simulink model "DrivetrainHevP2_SSC"  (R2022a)
settings: Solver=daessc  StartTime=0.0  StopTime=100  RelTol=1e-3
model workspace (MAT data in the model file):
  Aeff = 0.0314159265359
  Af = 2.27
  Apist_C0 = 0.0314159265359
  Apist_TCC = 0.001
  Bx = 10
  Cd = 0.25
  CoulFr_ShaftIn = 0
  Cx = 1.9
  DensAir = 1.293
  DerFac_C0 = 1
  DerFac_TCC = 1
  Drag_C0 = 0
  Drag_TCC = 0
  Dx = 1
  Eff_Diff = [0.98 0.98]
  Ex = 0.97
  FDrive = 3.32
  FZMAX = 6570
  FZMIN = 0
  G = [0 1 2 3 4 5 6]
  G_o = 1
  Iyy = 0.8
  Iyy_Whl = 0.8
  JCa_Diff = 0.001
  JEng = 0.01
  JMot = 0.21
  JPl_Diff = 0.001
  JShIn = 1e-05
  JShOut = 0.15
  Jd = 0.025
  Ji = 0.21
  Jin_Cltch = 0.2
  Jout = [0.009 0.01 0.01 0.01 0.01 0.01 0.01]
  Jout_Cltch = 0.01
  Jt = 0.01
  Jw1 = 0.01
  Jw2 = 0.01
  K_c = 10000
  KinFr_C0 = 0.4
  KinFr_TCC = 0.3
  Lrel = 0.15
  Mass = 1623
  N = [0.001 4.212 2.637 1.8 1.386 1 0.772]
  NF = 2
  NR = 2
  Ndiff = 3.32
  Ndisk = 1
  Neff_C0 = 1
  Neff_TCC = 6
  PEng_C0 = 30000
  PEng_TCC = 100
  Pabs = 101325
  Press = 300000
  PwrThr_Diff = [0.001 0.001]
  RatFr_ShaftIn = 1.1
  Re = 0.327
  Reff = 0.11
  Reff_C0 = 0.11
  Reff_TCC = 130
  Rm = 0.15
  SprStff_ShaftIn = 10000
  StatFr_C0 = 0.45
  StatFr_TCC = 0.35
  T = 273
  Temp_bpts = [313 358]
  Trq_bpts = [25 50 75 100 150 200 250]
  UNLOADED_RADIUS = 0.336
  VXLOW = 2
  VisFr_Diff = [0.001 0.001]
  ViscFr_ShaftIn = 400
  aMy = 0.01
  a_CG = 1.09
  alphaMy = 0
  b : Simulink.Parameter (value not decoded)
  bMy = 0
  b_CG = 1.7
  bd = 0.001
  betaMy = 1
  bi = 0.001
  bin_Cltch = 0.003
  bout = [0.003 0.003 0.003 0.003 0.003 0.003 0.003]
  bout_Cltch = 0.003
  br = 0.001
  bt = 0.001
  bw1 = 0.001
  bw2 = 0.001
  cMy = 0
  disk_abore = 0.05
  domega_o = 0
  eta = [0.95 0.95 0.95 0.95 0.95 0.95 0.95]
  eta_diff = 0.98
  eta_tbl = [1 1 1 1 1 1 1 1 1 1 1 1 ... (1078 elements, 7x11x7x2)]
  g = 9.81
  h = 0.5
  k : Simulink.Parameter (value not decoded)
  kappamax = 1.5
  lam_x = 1
  mu_kinetic = 0.35
  mu_static = 0.45
  muk = 0.4
  mus = 0.45
  num_pads = 2
  omega_bpts = [500.383141081 749.619781963 1002.67614148 1250.9578527 1499.23956393 1747.52127515 1995.80298637 2501.9157054 2998.47912785 4001.15526933 5003.83141081]
  omega_c : Simulink.Parameter (value not decoded)
  omega_o = 0
  omegai_o = 0
  omegal = 94.2477796077
  omegao = 0
  omegat_o = 0
  omegau = 83.7758040957
  omegaw1o = 0
  omegaw2o = 0
  phi = [0 0.5 0.6 0.7 0.8 0.87 0.92 0.94 0.96 0.97]
  phi_new = [0 0.5 0.6 0.7 0.8 0.87 0.92 0.94 0.96 0.97 0.99 1.02 ... (16 elements, 1x16)]
  philu = 0.85
  press = 700000
  psi = [12.2938 12.8588 13.1452 13.6285 14.6163 16.2675 19.3503 22.1046 29.9986 50]
  psi_new = [12.2938 12.8588 13.1452 13.6285 14.6163 16.2675 19.3503 22.1046 29.9986 50 48 41.76 ... (16 elements, 1x16)]
  tauC = 0.25
  tauTC = 0.1
  tau_s = 0.1
  theta_o = 0
  wc = 10
  win_o = 0
  wout_o = 0
  x_o = 0
  xdot_o = 0
  zeta = [2.232 1.5462 1.4058 1.2746 1.1528 1.0732 1.0192 0.9983 0.9983 0.9983]
  zeta_new = [2.232 1.5462 1.4058 1.2746 1.1528 1.0732 1.0192 0.9983 0.9983 0.9983 0.979797979798 1.04382929642 ... (16 elements, 1x16)]
libraries: fl_lib x66, nesl_utility x40, sdl_lib x25, simulink x7, autolibpowerinfoutils x5
(part 2 of 3)

== system DrivetrainHevP2_SSC/Sensor3 ==
  DiffTQ : nesl_utility/PS-Simulink Converter  PhysicalDomain=network_engine_domain  SubClassName=ps_output  LeftPortType=input  RightPortType=output  PseudoPeriodic=off  Frequencies=[]  VectorFormat=1-D array  Unit=1  AffineConversion=off
      settings: SourceProductBaseCode=SS,PW,VE
  Ideal Rotational Motion Sensor : fl_lib/Mechanical/Mechanical Sensors/Ideal Rotational Motion Sensor  wrap_angle=simscape.enum.onoff.off  offset=0 rad
      settings: SourceProductBaseCode=PW,SS,VE
  Ideal Torque Sensor : fl_lib/Mechanical/Mechanical Sensors/Ideal Torque Sensor
      settings: SourceProductBaseCode=PW,SS,VE
  Mechanical Rotational Reference : fl_lib/Mechanical/Rotational Elements/Mechanical Rotational Reference
      settings: SourceProductBaseCode=PW,SS,VE
  PS Terminator : fl_lib/Physical Signals/Sinks/PS Terminator
      settings: SourceProductBaseCode=PW,SS,VE
  PS-Simulink Converter : nesl_utility/PS-Simulink Converter  PhysicalDomain=network_engine_domain  SubClassName=ps_output  LeftPortType=input  RightPortType=output  PseudoPeriodic=off  Frequencies=[]  VectorFormat=1-D array  Unit=inherit  AffineConversion=off
      settings: SourceProductBaseCode=SS,PW,VE
  R : PMIOPort  Side=Left
  C : PMIOPort  Port=2  Side=Right
  Trq : Outport
  Spd : Outport  Port=2
  wires:
  DiffTQ/1 -> Trq/1
  PS-Simulink Converter/1 -> Spd/1
  connections:
  DiffTQ/LConn1 -- Ideal Torque Sensor/RConn2
  Ideal Torque Sensor/RConn1 -- C/RConn1
  Ideal Torque Sensor/LConn1 -- R/RConn1 -- Ideal Rotational Motion Sensor/LConn1
  PS Terminator/LConn1 -- Ideal Rotational Motion Sensor/RConn3
  PS-Simulink Converter/LConn1 -- Ideal Rotational Motion Sensor/RConn2
  Mechanical Rotational Reference/LConn1 -- Ideal Rotational Motion Sensor/RConn1

== system DrivetrainHevP2_SSC/Sensor4 ==
  Force : nesl_utility/PS-Simulink Converter  PhysicalDomain=network_engine_domain  SubClassName=ps_output  LeftPortType=input  RightPortType=output  PseudoPeriodic=off  Frequencies=[]  VectorFormat=1-D array  Unit=1  AffineConversion=off
      settings: SourceProductBaseCode=SS,PW,VE
  Ideal Force Sensor : fl_lib/Mechanical/Mechanical Sensors/Ideal Force Sensor
      settings: SourceProductBaseCode=PW,SS,VE
  Ideal Translational Motion Sensor : fl_lib/Mechanical/Mechanical Sensors/Ideal Translational Motion Sensor  offset=0 m
      settings: SourceProductBaseCode=PW,SS,VE
  Mechanical Translational Reference : fl_lib/Mechanical/Translational Elements/Mechanical Translational Reference
      settings: SourceProductBaseCode=PW,SS,VE
  SPD : nesl_utility/PS-Simulink Converter  PhysicalDomain=network_engine_domain  SubClassName=ps_output  LeftPortType=input  RightPortType=output  PseudoPeriodic=off  Frequencies=[]  VectorFormat=1-D array  Unit=1  AffineConversion=off
      settings: SourceProductBaseCode=SS,PW,VE
  Out : PMIOPort  Side=Left
  H : PMIOPort  Port=2  Side=Right
  VEVspd : Outport
  VEHforce : Outport  Port=2
  wires:
  Force/1 -> VEHforce/1
  SPD/1 -> VEVspd/1
  connections:
  Ideal Force Sensor/RConn1 -- Out/RConn1
  Ideal Force Sensor/RConn2 -- Force/LConn1
  SPD/LConn1 -- Ideal Translational Motion Sensor/RConn2
  Ideal Force Sensor/LConn1 -- Ideal Translational Motion Sensor/LConn1 -- H/RConn1
  Mechanical Translational Reference/LConn1 -- Ideal Translational Motion Sensor/RConn1

== system DrivetrainHevP2_SSC/Torque Converter and Lockup Clutch ==
  MtrTrq : Inport
  ClutchTrq : Inport  Port=2
  ClutchSpd : Inport  Port=3
  MtrSpd : Inport  Port=4
  TurbTrq : Inport  Port=5
  TurbSpd : Inport  Port=6
  Power Accounting Bus Creator2 : autolibpowerinfoutils/Power Accounting Bus Creator  AssctBlkSelPopup=Parent  RefBlkName='diff'  PwrTrnsfrdCheckBox=on  PwrNotTrnsfrdCheckBox=on  PwrStoredCheckBox=on  aMode=aMode
      settings: SourceProductBaseCode=PW,DR,MT,VE
  PwrAccountingDiff : Subsystem
  Terminator5 : Terminator
  wires:
  TurbTrq/1 -> PwrAccountingDiff/3(TurbTrq)
  TurbSpd/1 -> PwrAccountingDiff/5(TurbSpd)
  MtrTrq/1 -> PwrAccountingDiff/4(MtrTrq)
  ClutchTrq/1 -> PwrAccountingDiff/2(ClutchTrq)
  PwrAccountingDiff/3(PWRstored) -> Power Accounting Bus Creator2/3
  PwrAccountingDiff/1(PwrTrnsfrd) -> Power Accounting Bus Creator2/1
  PwrAccountingDiff/2(PwrNotTrnsfrd) -> Power Accounting Bus Creator2/2
  Power Accounting Bus Creator2/1 -> Terminator5/1
  ClutchSpd/1 -> PwrAccountingDiff/1(ClutchSpd)
  MtrSpd/1 -> PwrAccountingDiff/6(MtrSpd)

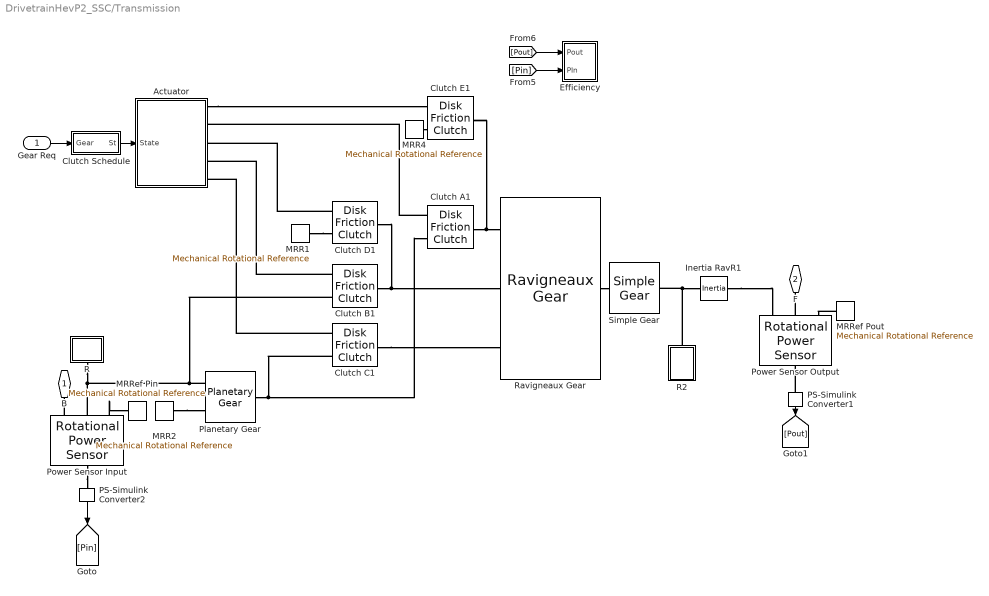
== system DrivetrainHevP2_SSC/Transmission ==
  Gear Req : Inport
  Actuator : Subsystem
  Clutch Schedule : Subsystem
  Clutch A1 : sdl_lib/Clutches/Disk Friction Clutch  geometry_model=sdl.enum.friction_geometry.annular  r_eff=130 mm  d_o=150 mm  d_i=100 mm  nS=6  piston_area=0.001 m^2  unidirectional=sdl.enum.directionality.bidirectional  friction_model=sdl.enum.friction_model_TLU_thermal.fixed  mu_w_vector=[ 0 0.1 0.2 0.3 0.4 0.5 1 2 5 10 100 1000 ] rad/s  temperature_TLU=[280.0, 300.0, 320.0] K  mu_static=0.65  mu_static_vector=[0.4, 0.38, 0.36]  mu_coulomb=0.6  mu_coulomb_vector=[ 0.29 0.28 0.26 0.22 0.21 0.2 0.2 0.19 0.19 0.19 0.19 0.19 ]  mu_coulomb_temp_vector=[0.3, 0.28, 0.25]  mu_coulomb_matrix=[0.34, 0.32, 0.3; 0.3, 0.28, 0.25; 0.25, 0.2, 0.15]  mu_interp_method=simscape.enum.interpolation.linear  mu_extrap_method=simscape.enum.extrapolation.linear  d_f=1  w_tol=0.001 rad/s  pressure_min=100 Pa  mu_visc=0 N*m/(rad/s)  initial_state_locked=sdl.enum.initial_lock.locked  enable_faults=simscape.enum.onoff.off  fault_type=sdl.enum.clutchFault.lock  external_fault=simscape.enum.onoff.off  temporal_fault=simscape.enum.onoff.off  fault_time=5 s  report_fault=simscape.enum.assert.action.none  thermal_mass=25 kJ/K  T_init=300 K
      settings: SourceProductBaseCode=LD  InternalSimscapePortConfiguration="{\"Bottom\":[],\"Left\":[{\"id\":\"P\",\"label\":\"P\",\"type\":\"input\"},{\"id\":\"B\",\"label\":\"B\",\"type\":\"foundation.mechanical.rotational.rotational\"}],\"Right\":[{\"id\":\"F\",\"label\":\"F\",\"type\":\"foundation.mechanical.rotational.rotational\"}],\"Top\":[]}"
  Clutch B1 : sdl_lib/Clutches/Disk Friction Clutch  geometry_model=sdl.enum.friction_geometry.annular  r_eff=130 mm  d_o=150 mm  d_i=100 mm  nS=6  piston_area=0.001 m^2  unidirectional=sdl.enum.directionality.bidirectional  friction_model=sdl.enum.friction_model_TLU_thermal.fixed  mu_w_vector=[ 0 0.1 0.2 0.3 0.4 0.5 1 2 5 10 100 1000 ] rad/s  temperature_TLU=[280.0, 300.0, 320.0] K  mu_static=0.65  mu_static_vector=[0.4, 0.38, 0.36]  mu_coulomb=0.6  mu_coulomb_vector=[ 0.29 0.28 0.26 0.22 0.21 0.2 0.2 0.19 0.19 0.19 0.19 0.19 ]  mu_coulomb_temp_vector=[0.3, 0.28, 0.25]  mu_coulomb_matrix=[0.34, 0.32, 0.3; 0.3, 0.28, 0.25; 0.25, 0.2, 0.15]  mu_interp_method=simscape.enum.interpolation.linear  mu_extrap_method=simscape.enum.extrapolation.linear  d_f=1  w_tol=0.001 rad/s  pressure_min=100 Pa  mu_visc=0 N*m/(rad/s)  initial_state_locked=sdl.enum.initial_lock.unlocked  enable_faults=simscape.enum.onoff.off  fault_type=sdl.enum.clutchFault.lock  external_fault=simscape.enum.onoff.off  temporal_fault=simscape.enum.onoff.off  fault_time=5 s  report_fault=simscape.enum.assert.action.none  thermal_mass=25 kJ/K  T_init=300 K
      settings: SourceProductBaseCode=LD  InternalSimscapePortConfiguration="{\"Bottom\":[],\"Left\":[{\"id\":\"P\",\"label\":\"P\",\"type\":\"input\"},{\"id\":\"B\",\"label\":\"B\",\"type\":\"foundation.mechanical.rotational.rotational\"}],\"Right\":[{\"id\":\"F\",\"label\":\"F\",\"type\":\"foundation.mechanical.rotational.rotational\"}],\"Top\":[]}"
  Clutch C1 : sdl_lib/Clutches/Disk Friction Clutch  geometry_model=sdl.enum.friction_geometry.annular  r_eff=130 mm  d_o=150 mm  d_i=100 mm  nS=6  piston_area=0.001 m^2  unidirectional=sdl.enum.directionality.bidirectional  friction_model=sdl.enum.friction_model_TLU_thermal.fixed  mu_w_vector=[ 0 0.1 0.2 0.3 0.4 0.5 1 2 5 10 100 1000 ] rad/s  temperature_TLU=[280.0, 300.0, 320.0] K  mu_static=0.65  mu_static_vector=[0.4, 0.38, 0.36]  mu_coulomb=0.6  mu_coulomb_vector=[ 0.29 0.28 0.26 0.22 0.21 0.2 0.2 0.19 0.19 0.19 0.19 0.19 ]  mu_coulomb_temp_vector=[0.3, 0.28, 0.25]  mu_coulomb_matrix=[0.34, 0.32, 0.3; 0.3, 0.28, 0.25; 0.25, 0.2, 0.15]  mu_interp_method=simscape.enum.interpolation.linear  mu_extrap_method=simscape.enum.extrapolation.linear  d_f=1  w_tol=0.001 rad/s  pressure_min=100 Pa  mu_visc=0 N*m/(rad/s)  initial_state_locked=sdl.enum.initial_lock.unlocked  enable_faults=simscape.enum.onoff.off  fault_type=sdl.enum.clutchFault.lock  external_fault=simscape.enum.onoff.off  temporal_fault=simscape.enum.onoff.off  fault_time=5 s  report_fault=simscape.enum.assert.action.none  thermal_mass=25 kJ/K  T_init=300 K
      settings: SourceProductBaseCode=LD  InternalSimscapePortConfiguration="{\"Bottom\":[],\"Left\":[{\"id\":\"P\",\"label\":\"P\",\"type\":\"input\"},{\"id\":\"B\",\"label\":\"B\",\"type\":\"foundation.mechanical.rotational.rotational\"}],\"Right\":[{\"id\":\"F\",\"label\":\"F\",\"type\":\"foundation.mechanical.rotational.rotational\"}],\"Top\":[]}"
  Clutch D1 : sdl_lib/Clutches/Disk Friction Clutch  geometry_model=sdl.enum.friction_geometry.annular  r_eff=130 mm  d_o=150 mm  d_i=100 mm  nS=6  piston_area=0.001 m^2  unidirectional=sdl.enum.directionality.bidirectional  friction_model=sdl.enum.friction_model_TLU_thermal.fixed  mu_w_vector=[ 0 0.1 0.2 0.3 0.4 0.5 1 2 5 10 100 1000 ] rad/s  temperature_TLU=[280.0, 300.0, 320.0] K  mu_static=0.65  mu_static_vector=[0.4, 0.38, 0.36]  mu_coulomb=0.6  mu_coulomb_vector=[ 0.29 0.28 0.26 0.22 0.21 0.2 0.2 0.19 0.19 0.19 0.19 0.19 ]  mu_coulomb_temp_vector=[0.3, 0.28, 0.25]  mu_coulomb_matrix=[0.34, 0.32, 0.3; 0.3, 0.28, 0.25; 0.25, 0.2, 0.15]  mu_interp_method=simscape.enum.interpolation.linear  mu_extrap_method=simscape.enum.extrapolation.linear  d_f=1  w_tol=0.001 rad/s  pressure_min=100 Pa  mu_visc=0 N*m/(rad/s)  initial_state_locked=sdl.enum.initial_lock.locked  enable_faults=simscape.enum.onoff.off  fault_type=sdl.enum.clutchFault.lock  external_fault=simscape.enum.onoff.off  temporal_fault=simscape.enum.onoff.off  fault_time=5 s  report_fault=simscape.enum.assert.action.none  thermal_mass=25 kJ/K  T_init=300 K
      settings: SourceProductBaseCode=LD  InternalSimscapePortConfiguration="{\"Bottom\":[],\"Left\":[{\"id\":\"P\",\"label\":\"P\",\"type\":\"input\"},{\"id\":\"B\",\"label\":\"B\",\"type\":\"foundation.mechanical.rotational.rotational\"}],\"Right\":[{\"id\":\"F\",\"label\":\"F\",\"type\":\"foundation.mechanical.rotational.rotational\"}],\"Top\":[]}"
  Clutch E1 : sdl_lib/Clutches/Disk Friction Clutch  geometry_model=sdl.enum.friction_geometry.annular  r_eff=130 mm  d_o=150 mm  d_i=100 mm  nS=6  piston_area=0.001 m^2  unidirectional=sdl.enum.directionality.bidirectional  friction_model=sdl.enum.friction_model_TLU_thermal.fixed  mu_w_vector=[ 0 0.1 0.2 0.3 0.4 0.5 1 2 5 10 100 1000 ] rad/s  temperature_TLU=[280.0, 300.0, 320.0] K  mu_static=0.65  mu_static_vector=[0.4, 0.38, 0.36]  mu_coulomb=0.6  mu_coulomb_vector=[ 0.29 0.28 0.26 0.22 0.21 0.2 0.2 0.19 0.19 0.19 0.19 0.19 ]  mu_coulomb_temp_vector=[0.3, 0.28, 0.25]  mu_coulomb_matrix=[0.34, 0.32, 0.3; 0.3, 0.28, 0.25; 0.25, 0.2, 0.15]  mu_interp_method=simscape.enum.interpolation.linear  mu_extrap_method=simscape.enum.extrapolation.linear  d_f=1  w_tol=0.001 rad/s  pressure_min=100 Pa  mu_visc=0 N*m/(rad/s)  initial_state_locked=sdl.enum.initial_lock.unlocked  enable_faults=simscape.enum.onoff.off  fault_type=sdl.enum.clutchFault.lock  external_fault=simscape.enum.onoff.off  temporal_fault=simscape.enum.onoff.off  fault_time=5 s  report_fault=simscape.enum.assert.action.none  thermal_mass=25 kJ/K  T_init=300 K
      settings: SourceProductBaseCode=LD  InternalSimscapePortConfiguration="{\"Bottom\":[],\"Left\":[{\"id\":\"P\",\"label\":\"P\",\"type\":\"input\"},{\"id\":\"B\",\"label\":\"B\",\"type\":\"foundation.mechanical.rotational.rotational\"}],\"Right\":[{\"id\":\"F\",\"label\":\"F\",\"type\":\"foundation.mechanical.rotational.rotational\"}],\"Top\":[]}"
  Efficiency : Subsystem
  Inertia RavR1 : fl_lib/Mechanical/Rotational Elements/Inertia  inertia=0.01 kg*m^2  num_ports=foundation.enum.numPorts2.two  w_specify=on  w_priority=High  w=0 rad/s  w_nominal_specify=off  w_nominal_unit=rad/s  w_nominal_value=1  t_specify=off  t_priority=High  t=0 N*m  t_nominal_specify=off  t_nominal_unit=N*m  t_nominal_value=1
      settings: SourceProductBaseCode=PW,SS,VE  InternalSimscapePortConfiguration="{\"Bottom\":[],\"Left\":[{\"id\":\"I\",\"label\":\"\",\"type\":\"foundation.mechanical.rotational.rotational\"}],\"Right\":[{\"id\":\"J\",\"label\":\"\",\"type\":\"foundation.mechanical.rotational.rotational\"}],\"Top\":[]}"
  MRR1 : fl_lib/Mechanical/Rotational Elements/Mechanical Rotational Reference
      settings: SourceProductBaseCode=PW,SS,VE
  MRR2 : fl_lib/Mechanical/Rotational Elements/Mechanical Rotational Reference
      settings: SourceProductBaseCode=PW,SS,VE
  MRR4 : fl_lib/Mechanical/Rotational Elements/Mechanical Rotational Reference
      settings: SourceProductBaseCode=PW,SS,VE
  MRRef Pin : fl_lib/Mechanical/Rotational Elements/Mechanical Rotational Reference
      settings: SourceProductBaseCode=PW,SS,VE
  MRRef Pout : fl_lib/Mechanical/Rotational Elements/Mechanical Rotational Reference
      settings: SourceProductBaseCode=PW,SS,VE
  PS-Simulink Converter1 : nesl_utility/PS-Simulink Converter  PhysicalDomain=network_engine_domain  SubClassName=ps_output  LeftPortType=input  RightPortType=output  PseudoPeriodic=off  Frequencies=[]  VectorFormat=1-D array  Unit=HP_DIN  AffineConversion=off
      settings: SourceProductBaseCode=SS,PW,VE
  PS-Simulink Converter2 : nesl_utility/PS-Simulink Converter  PhysicalDomain=network_engine_domain  SubClassName=ps_output  LeftPortType=input  RightPortType=output  PseudoPeriodic=off  Frequencies=[]  VectorFormat=1-D array  Unit=HP_DIN  AffineConversion=off
      settings: SourceProductBaseCode=SS,PW,VE
  Planetary Gear : sdl_lib/Gears/Planetary Gear  rs_ratio=1.92424631  friction_model=sdl.enum.gear_friction.constant  efficiency=[ 0.95 0.95]  temperature_TLU=[ 280 300 320 ] K  efficiency_sp_TLU=[ 0.95 0.9 0.85 ]  efficiency_rp_TLU=[ 0.95 0.9 0.85 ]  pwr_thr=[ 0.001 0.001 ] W  mu_visc=[ 0 0 ] N*m/(rad/s)  model_inertia=simscape.enum.onoff.on  planet_inertia=0.001 kg*m^2  thermal_mass=50 J/K  T_init=300 K
      settings: SourceProductBaseCode=LD
  Power Sensor Input : sdl_lib/Sensors/Rotational Power Sensor  measurement_type=1  averaging_period=1 s  max_frequency=1000 Hz  max_speed=1000 rpm
      settings: SourceProductBaseCode=LD  InternalSimscapePortConfiguration="{\"Bottom\":[],\"Left\":[{\"id\":\"S\",\"label\":\"S\",\"type\":\"foundation.mechanical.rotational.rotational\"},{\"id\":\"R\",\"label\":\"R\",\"type\":\"foundation.mechanical.rotational.rotational\"},{\"id\":\"C\",\"label\":\"C\",\"type\":\"foundation.mechanical.rotational.rotational\"}],\"Right\":[{\"id\":\"P\",\"label\":\"P\",\"type\":\"output\"}],\"Top\":[]}"
  Power Sensor Output : sdl_lib/Sensors/Rotational Power Sensor  measurement_type=1  averaging_period=1 s  max_frequency=1000 Hz  max_speed=1000 rpm
      settings: SourceProductBaseCode=LD  InternalSimscapePortConfiguration="{\"Bottom\":[],\"Left\":[{\"id\":\"S\",\"label\":\"S\",\"type\":\"foundation.mechanical.rotational.rotational\"},{\"id\":\"R\",\"label\":\"R\",\"type\":\"foundation.mechanical.rotational.rotational\"},{\"id\":\"C\",\"label\":\"C\",\"type\":\"foundation.mechanical.rotational.rotational\"}],\"Right\":[{\"id\":\"P\",\"label\":\"P\",\"type\":\"output\"}],\"Top\":[]}"
  R : Subsystem
  R2 : Subsystem
  Ravigneaux Gear : sdl_lib/Gears/Ravigneaux Gear  rsl_ratio=1.85391061211  rss_ratio=2.3400145  friction_model=sdl.enum.gear_friction.constant  efficiency=[ 0.95 0.95 0.95 0.95 ]  temperature_TLU=[ 280 300 320 ] K  efficiency_lsp_TLU=[ 0.95 0.9 0.85 ]  efficiency_ssp_TLU=[ 0.95 0.9 0.85 ]  efficiency_rp_TLU=[ 0.95 0.9 0.85 ]  efficiency_pp_TLU=[ 0.95 0.9 0.85 ]  pwr_thr=[ 0.001 0.001 0.001 0.001 ] W  mu_visc=[ 0 0 0 0 ] N*m/(rad/s)  model_inertia=simscape.enum.onoff.on  inner_planet_inertia=0.001 kg*m^2  outer_planet_inertia=0.001 kg*m^2  thermal_mass=50 J/K  T_init=300 K
      settings: SourceProductBaseCode=LD  InternalSimscapePortConfiguration="{\"Bottom\":[],\"Left\":[{\"id\":\"SL\",\"label\":\"SL\",\"type\":\"foundation.mechanical.rotational.rotational\"},{\"id\":\"C\",\"label\":\"C\",\"type\":\"foundation.mechanical.rotational.rotational\"},{\"id\":\"SS\",\"label\":\"SS\",\"type\":\"foundation.mechanical.rotational.rotational\"}],\"Right\":[{\"id\":\"R\",\"label\":\"R\",\"type\":\"foundation.mechanical.rotational.rotational\"}],\"Top\":[]}"
  Simple Gear : sdl_lib/Gears/Simple Gear  ratio=1.1844541232  rotation_direction=sdl.enum.shaftOutputDirection.same  friction_model=sdl.enum.gear_efficiencies_load.constant  T_noload=0.1 N*m  T_nom=5 N*m  efficiency_nom=0.8  efficiency=.95  temperature_TLU=[280, 300, 320] K  load_TLU=[1, 5, 10] N*m  efficiency_TLU=[.95, .9, .85]  efficiency_TLU2=[.85, .8, .75; .95, .9, .85; .85, .8, .7]  w_thr=0.01 rad/s  pwr_thr=0.001 W  backlash_model=sdl.enum.backlashModel.Off  backlash_distance=1e-3 mm  x0=0 m  r_base=0.1 m  hardstop_model=simscape.enum.hardstop.smooth  transition=1e-4 mm  backlash_stiffness=1e7 N/m  backlash_damping=1e6 N/(m/s)  e=0  v_tol=0.001 m/s  mu_visc=[0, 0] N*m/(rad/s)  enable_faults=simscape.enum.onoff.off  efficiency_fault=0.05  external_fault=simscape.enum.onoff.off  temporal_fault=simscape.enum.onoff.off  fault_time=5 s  fault_angles=pi / 12 rad  report_fault=simscape.enum.assert.action.none  thermal_mass=50 J/K  temperature_specify=off  temperature_priority=High  temperature=300 K  temperature_nominal_specify=off  temperature_nominal_unit=K  temperature_nominal_value=1  x_backlash_specify=off  x_backlash_priority=None  x_backlash=0 mm  x_backlash_nominal_specify=off  x_backlash_nominal_unit=mm  x_backlash_nominal_value=1  f_hardstop_specify=off  f_hardstop_priority=None  f_hardstop=0 N  f_hardstop_nominal_specify=off  f_hardstop_nominal_unit=N  f_hardstop_nominal_value=1  v_backlash_specify=off  v_backlash_priority=None  v_backlash=0 m/s  v_backlash_nominal_specify=off  v_backlash_nominal_unit=m/s  v_backlash_nominal_value=1
  B : PMIOPort  Side=Left
  F : PMIOPort  Port=2  Side=Right
  wires:
  Gear Req/1 -> Clutch Schedule/1(Gear)
  PS-Simulink Converter2/1 -> [Pin]
  PS-Simulink Converter1/1 -> [Pout]
  Clutch Schedule/1(St) -> Actuator/1(State)
  [Pout] -> Efficiency/1(Pout)
  [Pin] -> Efficiency/2(PIn)
  connections:
  Power Sensor Output/LConn2 -- F/RConn1
  Power Sensor Input/LConn1 -- B/RConn1
  PS-Simulink Converter1/LConn1 -- Power Sensor Output/RConn1
  MRRef Pout/LConn1 -- Power Sensor Output/LConn3
  Power Sensor Input/RConn1 -- PS-Simulink Converter2/LConn1
  Power Sensor Input/LConn3 -- MRRef Pin/LConn1
  Inertia RavR1/RConn1 -- Power Sensor Output/LConn1
  R2/LConn1 -- Simple Gear/RConn1 -- Inertia RavR1/LConn1
  Clutch B1/LConn1 -- Actuator/RConn4
  Clutch C1/LConn1 -- Actuator/RConn5
  Clutch A1/LConn1 -- Actuator/RConn2
  Clutch D1/LConn1 -- Actuator/RConn3
  Actuator/RConn1 -- Clutch E1/LConn1
  Clutch A1/RConn1 -- Clutch E1/RConn1 -- Ravigneaux Gear/LConn1
  Clutch C1/LConn2 -- Clutch A1/LConn2 -- Planetary Gear/LConn1
  MRR2/LConn1 -- Planetary Gear/RConn2
  Ravigneaux Gear/RConn1 -- Simple Gear/LConn1
  Clutch C1/RConn1 -- Ravigneaux Gear/LConn3
  Clutch B1/LConn2 -- Power Sensor Input/LConn2 -- R/LConn1 -- Planetary Gear/RConn1
  MRR1/LConn1 -- Clutch D1/LConn2
  Clutch D1/RConn1 -- Clutch B1/RConn1 -- Ravigneaux Gear/LConn2
  MRR4/LConn1 -- Clutch E1/LConn2

== system DrivetrainHevP2_SSC/Vehicle ==
  FLaxleTQ : Inport
  FLaxleSPD : Inport  Port=2
  FRaxleTQ : Inport  Port=3
  FRaxleSPD : Inport  Port=4
  RLaxleTQ : Inport  Port=5
  RLaxleSPD : Inport  Port=6
  RRaxleTQ : Inport  Port=7
  RRaxleSPD : Inport  Port=8
  Vforce : Inport  Port=9
  Vspd : Inport  Port=10
  Power Accounting Bus Creator1 : autolibpowerinfoutils/Power Accounting Bus Creator  AssctBlkSelPopup=Parent  RefBlkName='diff'  PwrTrnsfrdCheckBox=on  PwrNotTrnsfrdCheckBox=on  PwrStoredCheckBox=on  aMode=aMode
      settings: SourceProductBaseCode=PW,DR,MT,VE
  PowerAccountingVEH : Subsystem
  Terminator1 : Terminator
  wires:
  RRaxleTQ/1 -> PowerAccountingVEH/7(RRaxleTQ)
  FRaxleSPD/1 -> PowerAccountingVEH/4(FRaxleSPD)
  FRaxleTQ/1 -> PowerAccountingVEH/3(FRaxleTQ)
  PowerAccountingVEH/1(PwrTrnsfrd) -> Power Accounting Bus Creator1/1
  RRaxleSPD/1 -> PowerAccountingVEH/8(RRaxleSPD)
  PowerAccountingVEH/3(PWRstored) -> Power Accounting Bus Creator1/3
  Vspd/1 -> PowerAccountingVEH/10(Vspd)
  FLaxleSPD/1 -> PowerAccountingVEH/2(FLaxleSPD)
  RLaxleTQ/1 -> PowerAccountingVEH/5(RLaxleTQ)
  Power Accounting Bus Creator1/1 -> Terminator1/1
  Vforce/1 -> PowerAccountingVEH/9(Vforce)
  FLaxleTQ/1 -> PowerAccountingVEH/1(FLaxleTQ)
  RLaxleSPD/1 -> PowerAccountingVEH/6(RLaxleSPD)
  PowerAccountingVEH/2(PwrNotTrnsfrd) -> Power Accounting Bus Creator1/2

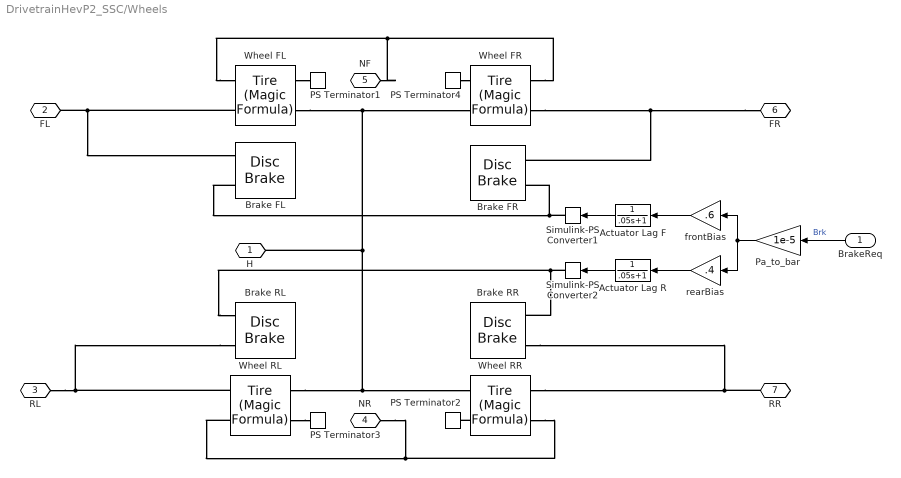
== system DrivetrainHevP2_SSC/Wheels ==
  BrakeReq : Inport
  Actuator Lag F : TransferFcn  Denominator=[.05 1]
  Actuator Lag R : TransferFcn  Denominator=[.05 1]
  Brake FL : sdl_lib/Brakes & Detents/Rotational/Disc Brake  r_mean=Rm m  bore=disk_abore m  n_pads=num_pads  thermal_port=simscape.enum.thermaleffects.omit  mu_static=mu_static  mu_coulomb=mu_kinetic  temperature_TLU=[280, 300, 320] K  mu_static_TLU=[.9, .8, .7]  mu_coulomb_TLU=[.8, .7, .6]  brkwy_vel=0.1 rad/s  visc_coef=0.001 N*m/(rad/s)  enable_faults=simscape.enum.onoff.off  faulted_pressure=0 bar  external_fault=simscape.enum.onoff.off  temporal_fault=simscape.enum.onoff.off  fault_time=5 s  report_fault=simscape.enum.assert.action.none  thermal_mass=50 kJ/K  temperature_specify=off  temperature_priority=High  temperature=300 K  temperature_nominal_specify=off  temperature_nominal_unit=K  temperature_nominal_value=1
      settings: SourceProductBaseCode=LD
  Brake FR : sdl_lib/Brakes & Detents/Rotational/Disc Brake  r_mean=Rm m  bore=disk_abore m  n_pads=num_pads  thermal_port=simscape.enum.thermaleffects.omit  mu_static=mu_static  mu_coulomb=mu_kinetic  temperature_TLU=[280, 300, 320] K  mu_static_TLU=[.9, .8, .7]  mu_coulomb_TLU=[.8, .7, .6]  brkwy_vel=0.1 rad/s  visc_coef=0.001 N*m/(rad/s)  enable_faults=simscape.enum.onoff.off  faulted_pressure=0 bar  external_fault=simscape.enum.onoff.off  temporal_fault=simscape.enum.onoff.off  fault_time=5 s  report_fault=simscape.enum.assert.action.none  thermal_mass=50 kJ/K  temperature_specify=off  temperature_priority=High  temperature=300 K  temperature_nominal_specify=off  temperature_nominal_unit=K  temperature_nominal_value=1
      settings: SourceProductBaseCode=LD
  Brake RL : sdl_lib/Brakes & Detents/Rotational/Disc Brake  r_mean=Rm m  bore=disk_abore m  n_pads=num_pads  thermal_port=simscape.enum.thermaleffects.omit  mu_static=mu_static  mu_coulomb=mu_kinetic  temperature_TLU=[280, 300, 320] K  mu_static_TLU=[.9, .8, .7]  mu_coulomb_TLU=[.8, .7, .6]  brkwy_vel=0.1 rad/s  visc_coef=0.001 N*m/(rad/s)  enable_faults=simscape.enum.onoff.off  faulted_pressure=0 bar  external_fault=simscape.enum.onoff.off  temporal_fault=simscape.enum.onoff.off  fault_time=5 s  report_fault=simscape.enum.assert.action.none  thermal_mass=50 kJ/K  temperature_specify=off  temperature_priority=High  temperature=300 K  temperature_nominal_specify=off  temperature_nominal_unit=K  temperature_nominal_value=1
      settings: SourceProductBaseCode=LD
  Brake RR : sdl_lib/Brakes & Detents/Rotational/Disc Brake  r_mean=Rm m  bore=disk_abore m  n_pads=num_pads  thermal_port=simscape.enum.thermaleffects.omit  mu_static=mu_static  mu_coulomb=mu_kinetic  temperature_TLU=[280, 300, 320] K  mu_static_TLU=[.9, .8, .7]  mu_coulomb_TLU=[.8, .7, .6]  brkwy_vel=0.1 rad/s  visc_coef=0.001 N*m/(rad/s)  enable_faults=simscape.enum.onoff.off  faulted_pressure=0 bar  external_fault=simscape.enum.onoff.off  temporal_fault=simscape.enum.onoff.off  fault_time=5 s  report_fault=simscape.enum.assert.action.none  thermal_mass=50 kJ/K  temperature_specify=off  temperature_priority=High  temperature=300 K  temperature_nominal_specify=off  temperature_nominal_unit=K  temperature_nominal_value=1
      settings: SourceProductBaseCode=LD
  PS Terminator{1..4} (4 alike) : fl_lib/Physical Signals/Sinks/PS Terminator
      settings: SourceProductBaseCode=PW,SS,VE
  Pa_to_bar : Gain  Gain=1e-5
  Simulink-PS Converter1 : nesl_utility/Simulink-PS Converter  PhysicalDomain=network_engine_domain  SubClassName=ps_input  LeftPortType=input  RightPortType=output  PseudoPeriodic=off  Frequencies=[]  NoiseDistribution=none  NoiseParameters=[]  Unit=bar  AffineConversion=off  FilteringAndDerivatives=provide  SimscapeFilterOrder=1  InputFilterTimeConstant=0.01  UdotUserProvided=0
      settings: SourceProductBaseCode=SS,PW,VE
  Simulink-PS Converter2 : nesl_utility/Simulink-PS Converter  PhysicalDomain=network_engine_domain  SubClassName=ps_input  LeftPortType=input  RightPortType=output  PseudoPeriodic=off  Frequencies=[]  NoiseDistribution=none  NoiseParameters=[]  Unit=bar  AffineConversion=off  FilteringAndDerivatives=provide  SimscapeFilterOrder=1  InputFilterTimeConstant=0.01  UdotUserProvided=0
      settings: SourceProductBaseCode=SS,PW,VE
  Wheel FL : sdl_lib/Tires & Vehicles/Tire (Magic Formula)  parameterization=sdl.enum.magic_tire_model.constant  F_z1=4000 N  F_x1=5000 N  kappa1=kappamax  B_m=Bx  C_m=Cx  D_m=Dx  E_m=Ex  fz0=4000 N  p_Cx=1.685  p_Dx=[1.21, -.037]  p_Ex=[.344, .095, -.02, 0]  p_Kx=[21.51, -.163, .245]  p_Hx=[-.002, .002]  p_Vx=[0, 0]  r_e=Re m  model_compliance=0  stiffness=1e6 N/m  damping=1000 N/(m/s)  model_inertia=1  inertia=Iyy kg*m^2  initial_velocity=0 rad/s  model_resistance=1  resistance_model=2  coeff=aMy  p_tire=press Pa  alpha=alphaMy  beta=betaMy  coeff_a=aMy  coeff_b=bMy s/m  coeff_c=cMy s^2/m^2  v_thr=0.001 m/s  v_tr_thr=VXLOW m/s
  Wheel FR : sdl_lib/Tires & Vehicles/Tire (Magic Formula)  parameterization=sdl.enum.magic_tire_model.constant  F_z1=4000 N  F_x1=5000 N  kappa1=kappamax  B_m=Bx  C_m=Cx  D_m=Dx  E_m=Ex  fz0=4000 N  p_Cx=1.685  p_Dx=[1.21, -.037]  p_Ex=[.344, .095, -.02, 0]  p_Kx=[21.51, -.163, .245]  p_Hx=[-.002, .002]  p_Vx=[0, 0]  r_e=Re m  model_compliance=0  stiffness=1e6 N/m  damping=1000 N/(m/s)  model_inertia=1  inertia=Iyy kg*m^2  initial_velocity=0 rad/s  model_resistance=1  resistance_model=2  coeff=aMy  p_tire=press Pa  alpha=alphaMy  beta=betaMy  coeff_a=aMy  coeff_b=bMy s/m  coeff_c=cMy s^2/m^2  v_thr=0.001 m/s  v_tr_thr=VXLOW m/s
  Wheel RL : sdl_lib/Tires & Vehicles/Tire (Magic Formula)  parameterization=sdl.enum.magic_tire_model.constant  F_z1=4000 N  F_x1=5000 N  kappa1=kappamax  B_m=Bx  C_m=Cx  D_m=Dx  E_m=Ex  fz0=4000 N  p_Cx=1.685  p_Dx=[1.21, -.037]  p_Ex=[.344, .095, -.02, 0]  p_Kx=[21.51, -.163, .245]  p_Hx=[-.002, .002]  p_Vx=[0, 0]  r_e=Re m  model_compliance=0  stiffness=1e6 N/m  damping=1000 N/(m/s)  model_inertia=1  inertia=Iyy kg*m^2  initial_velocity=0 rad/s  model_resistance=1  resistance_model=2  coeff=aMy  p_tire=press Pa  alpha=alphaMy  beta=betaMy  coeff_a=aMy  coeff_b=bMy s/m  coeff_c=cMy s^2/m^2  v_thr=0.001 m/s  v_tr_thr=VXLOW m/s
  Wheel RR : sdl_lib/Tires & Vehicles/Tire (Magic Formula)  parameterization=sdl.enum.magic_tire_model.constant  F_z1=4000 N  F_x1=5000 N  kappa1=kappamax  B_m=Bx  C_m=Cx  D_m=Dx  E_m=Ex  fz0=4000 N  p_Cx=1.685  p_Dx=[1.21, -.037]  p_Ex=[.344, .095, -.02, 0]  p_Kx=[21.51, -.163, .245]  p_Hx=[-.002, .002]  p_Vx=[0, 0]  r_e=Re m  model_compliance=0  stiffness=1e6 N/m  damping=1000 N/(m/s)  model_inertia=1  inertia=Iyy kg*m^2  initial_velocity=0 rad/s  model_resistance=1  resistance_model=2  coeff=aMy  p_tire=press Pa  alpha=alphaMy  beta=betaMy  coeff_a=aMy  coeff_b=bMy s/m  coeff_c=cMy s^2/m^2  v_thr=0.001 m/s  v_tr_thr=VXLOW m/s
  frontBias : Gain  Gain=.6
  rearBias : Gain  Gain=.4
  H : PMIOPort  Side=Left
  FL : PMIOPort  Port=2  Side=Left
  RL : PMIOPort  Port=3  Side=Left
  NR : PMIOPort  Port=4  Side=Left
  NF : PMIOPort  Port=5  Side=Left
  FR : PMIOPort  Port=6  Side=Right
  RR : PMIOPort  Port=7  Side=Right
  wires:
  BrakeReq/1 -> Pa_to_bar/1  "Brk"
  Actuator Lag R/1 -> Simulink-PS Converter2/1
  rearBias/1 -> Actuator Lag R/1
  frontBias/1 -> Actuator Lag F/1
  Pa_to_bar/1 -> frontBias/1, rearBias/1
  Actuator Lag F/1 -> Simulink-PS Converter1/1
  connections:
  FR/RConn1 -- Brake FR/LConn2 -- Wheel FR/LConn2
  Brake RR/LConn2 -- Wheel RR/LConn2 -- RR/RConn1
  Brake RL/LConn2 -- Wheel RL/LConn2 -- RL/RConn1
  Wheel FL/LConn2 -- Brake FL/LConn2 -- FL/RConn1
  H/RConn1 -- Wheel FL/RConn2 -- Wheel FR/RConn2 -- Wheel RR/RConn2 -- Wheel RL/RConn2
  Brake RL/LConn1 -- Brake RR/LConn1 -- Simulink-PS Converter2/RConn1
  Wheel FL/LConn1 -- Wheel FR/LConn1 -- NF/RConn1
  Wheel FL/RConn1 -- PS Terminator1/LConn1
  Wheel RR/LConn1 -- Wheel RL/LConn1 -- NR/RConn1
  PS Terminator4/LConn1 -- Wheel FR/RConn1
  Brake FR/LConn1 -- Brake FL/LConn1 -- Simulink-PS Converter1/RConn1
  Wheel RL/RConn1 -- PS Terminator3/LConn1
  Wheel RR/RConn1 -- PS Terminator2/LConn1

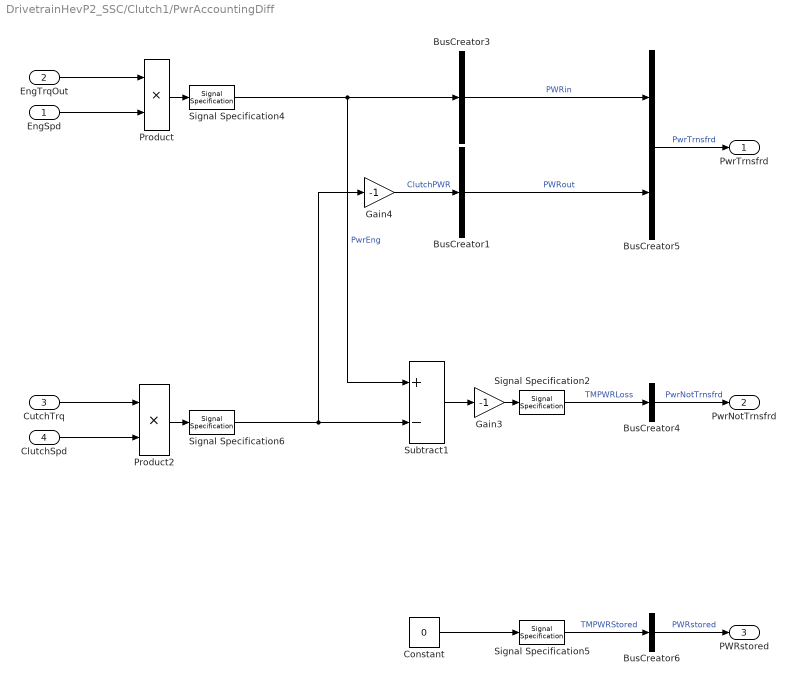
== system DrivetrainHevP2_SSC/Clutch1/PwrAccountingDiff ==
  EngSpd : Inport
  EngTrqOut : Inport  Port=2
  CutchTrq : Inport  Port=3
  ClutchSpd : Inport  Port=4
  BusCreator{1,3..4,6} (4 alike) : BusCreator  Inputs=1
  BusCreator5 : BusCreator  Inputs=2
  Constant : Constant  Value=0
  Gain3 : Gain  Gain=-1
  Gain4 : Gain  Gain=-1
  Product : Product
  Product2 : Product
  Signal Specification{2,4..6} (4 alike) : SignalSpecification  Unit=W
  Subtract1 : Sum  Inputs=+-
  PwrTrnsfrd : Outport
  PwrNotTrnsfrd : Outport  Port=2
  PWRstored : Outport  Port=3
  wires:
  Constant/1 -> Signal Specification5/1
  Product/1 -> Signal Specification4/1
  CutchTrq/1 -> Product2/1
  Product2/1 -> Signal Specification6/1
  Signal Specification2/1 -> BusCreator4/1  "TMPWRLoss"
  Gain3/1 -> Signal Specification2/1
  BusCreator3/1 -> BusCreator5/1  "PWRin"
  Signal Specification4/1 -> Subtract1/1, BusCreator3/1  "PwrEng"
  BusCreator1/1 -> BusCreator5/2  "PWRout"
  Signal Specification5/1 -> BusCreator6/1  "TMPWRStored"
  Signal Specification6/1 -> Gain4/1, Subtract1/2
  Subtract1/1 -> Gain3/1
  Gain4/1 -> BusCreator1/1  "ClutchPWR"
  BusCreator4/1 -> PwrNotTrnsfrd/1  "PwrNotTrnsfrd"
  ClutchSpd/1 -> Product2/2
  BusCreator6/1 -> PWRstored/1  "PWRstored"
  BusCreator5/1 -> PwrTrnsfrd/1  "PwrTrnsfrd"
  EngTrqOut/1 -> Product/1
  EngSpd/1 -> Product/2

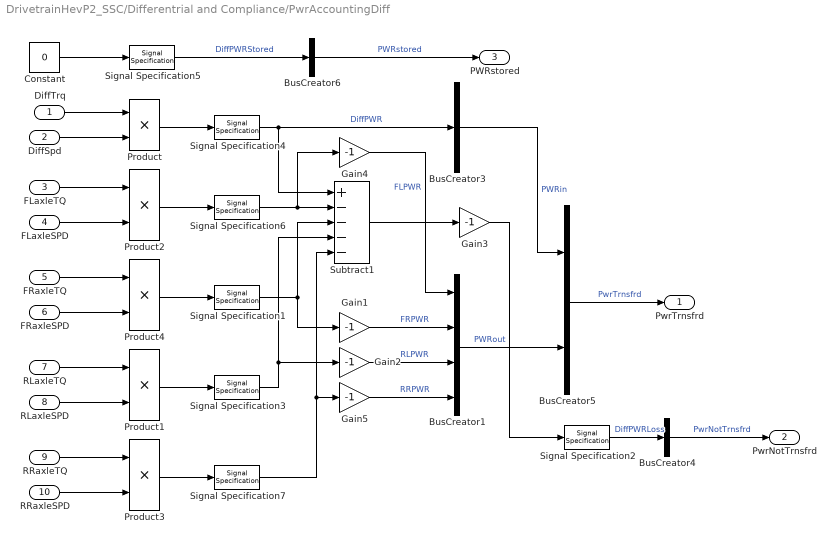
== system DrivetrainHevP2_SSC/Differentrial and Compliance/PwrAccountingDiff ==
  DiffTrq : Inport
  DiffSpd : Inport  Port=2
  FLaxleTQ : Inport  Port=3
  FLaxleSPD : Inport  Port=4
  FRaxleTQ : Inport  Port=5
  FRaxleSPD : Inport  Port=6
  RLaxleTQ : Inport  Port=7
  RLaxleSPD : Inport  Port=8
  RRaxleTQ : Inport  Port=9
  RRaxleSPD : Inport  Port=10
  BusCreator1 : BusCreator  Inputs=4
  BusCreator3 : BusCreator  Inputs=1
  BusCreator4 : BusCreator  Inputs=1
  BusCreator5 : BusCreator  Inputs=2
  BusCreator6 : BusCreator  Inputs=1
  Constant : Constant  Value=0
  Gain{1..5} (5 alike) : Gain  Gain=-1
  Product{,1..4} (5 alike) : Product
  Signal Specification{1..7} (7 alike) : SignalSpecification  Unit=W
  Subtract1 : Sum  Inputs=+----
  PwrTrnsfrd : Outport
  PwrNotTrnsfrd : Outport  Port=2
  PWRstored : Outport  Port=3
  wires:
  RRaxleTQ/1 -> Product3/1
  Gain5/1 -> BusCreator1/4  "RRPWR"
  RLaxleSPD/1 -> Product1/2
  Gain2/1 -> BusCreator1/3  "RLPWR"
  RRaxleSPD/1 -> Product3/2
  Product3/1 -> Signal Specification7/1
  Product1/1 -> Signal Specification3/1
  RLaxleTQ/1 -> Product1/1
  BusCreator4/1 -> PwrNotTrnsfrd/1  "PwrNotTrnsfrd"
  FLaxleTQ/1 -> Product2/1
  BusCreator5/1 -> PwrTrnsfrd/1  "PwrTrnsfrd"
  FRaxleTQ/1 -> Product4/1
  DiffSpd/1 -> Product/2
  BusCreator6/1 -> PWRstored/1  "PWRstored"
  Signal Specification1/1 -> Subtract1/3, Gain1/1
  Signal Specification5/1 -> BusCreator6/1  "DiffPWRStored"
  Subtract1/1 -> Gain3/1
  FRaxleSPD/1 -> Product4/2
  BusCreator1/1 -> BusCreator5/2  "PWRout"
  Gain4/1 -> BusCreator1/1  "FLPWR"
  Signal Specification2/1 -> BusCreator4/1  "DiffPWRLoss"
  FLaxleSPD/1 -> Product2/2
  BusCreator3/1 -> BusCreator5/1  "PWRin"
  Product2/1 -> Signal Specification6/1
  Gain1/1 -> BusCreator1/2  "FRPWR"
  Gain3/1 -> Signal Specification2/1
  Product4/1 -> Signal Specification1/1
  DiffTrq/1 -> Product/1
  Signal Specification7/1 -> Subtract1/5, Gain5/1
  Constant/1 -> Signal Specification5/1
  Product/1 -> Signal Specification4/1
  Signal Specification3/1 -> Subtract1/4, Gain2/1
  Signal Specification6/1 -> Subtract1/2, Gain4/1
  Signal Specification4/1 -> Subtract1/1, BusCreator3/1  "DiffPWR"

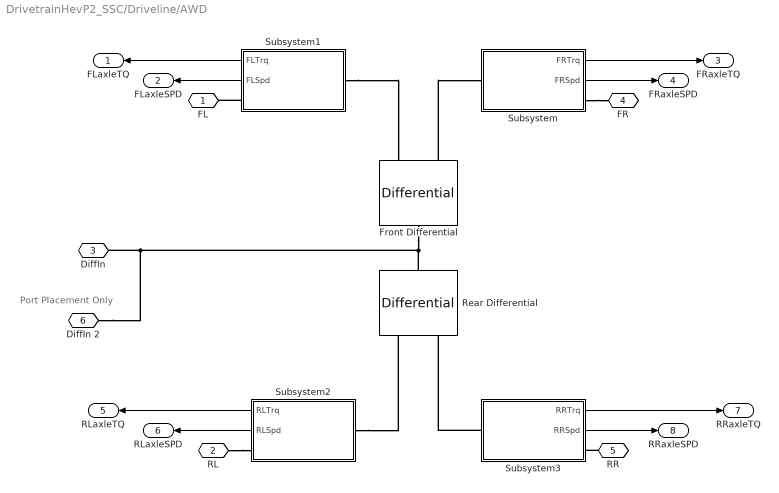
== system DrivetrainHevP2_SSC/Driveline/AWD ==
  note: Port Placement
      | Only
  Front Differential : sdl_lib/Gears/Differential  driveshaft_location=2  cd_ratio=FDrive  friction_model=2  efficiency=Eff_Diff  temperature_TLU=[ 280 300 320 ] K  efficiency_ss_TLU=[ 0.95 0.9 0.85 ]  efficiency_cd_TLU=[ 0.95 0.9 0.85 ]  pwr_thr=PwrThr_Diff W  mu_visc=VisFr_Diff N*m/(rad/s)  model_inertia=1  carrier_inertia=JCa_Diff kg*m^2  planet_inertia=JPl_Diff kg*m^2  thermal_mass=50 J/K  T_init=300 K
      settings: SourceProductBaseCode=LD
  Rear Differential : sdl_lib/Gears/Differential  driveshaft_location=2  cd_ratio=FDrive  friction_model=2  efficiency=Eff_Diff  temperature_TLU=[ 280 300 320 ] K  efficiency_ss_TLU=[ 0.95 0.9 0.85 ]  efficiency_cd_TLU=[ 0.95 0.9 0.85 ]  pwr_thr=PwrThr_Diff W  mu_visc=VisFr_Diff N*m/(rad/s)  model_inertia=1  carrier_inertia=JCa_Diff kg*m^2  planet_inertia=JPl_Diff kg*m^2  thermal_mass=50 J/K  T_init=300 K
      settings: SourceProductBaseCode=LD
  Subsystem : Subsystem
  Subsystem1 : Subsystem
  Subsystem2 : Subsystem
  Subsystem3 : Subsystem
  FL : PMIOPort  Side=Left
  RL : PMIOPort  Port=2  Side=Left
  DiffIn : PMIOPort  Port=3  Side=Left
  FR : PMIOPort  Port=4  Side=Right
  RR : PMIOPort  Port=5  Side=Right
  DiffIn 2 : PMIOPort  Port=6  Side=Right
  FLaxleTQ : Outport
  FLaxleSPD : Outport  Port=2
  FRaxleTQ : Outport  Port=3
  FRaxleSPD : Outport  Port=4
  RLaxleTQ : Outport  Port=5
  RLaxleSPD : Outport  Port=6
  RRaxleTQ : Outport  Port=7
  RRaxleSPD : Outport  Port=8
  wires:
  Subsystem1/2(FLSpd) -> FLaxleSPD/1
  Subsystem1/1(FLTrq) -> FLaxleTQ/1
  Subsystem/2(FRSpd) -> FRaxleSPD/1
  Subsystem/1(FRTrq) -> FRaxleTQ/1
  Subsystem2/1(RLTrq) -> RLaxleTQ/1
  Subsystem2/2(RLSpd) -> RLaxleSPD/1
  Subsystem3/1(RRTrq) -> RRaxleTQ/1
  Subsystem3/2(RRSpd) -> RRaxleSPD/1
  connections:
  Rear Differential/LConn1 -- DiffIn 2/RConn1 -- DiffIn/RConn1 -- Front Differential/LConn1
  Subsystem1/RConn1 -- FL/RConn1
  Subsystem3/LConn1 -- Rear Differential/RConn2
  RL/RConn1 -- Subsystem2/RConn1
  Subsystem1/LConn1 -- Front Differential/RConn1
  Subsystem/RConn1 -- FR/RConn1
  Front Differential/RConn2 -- Subsystem/LConn1
  Subsystem2/LConn1 -- Rear Differential/RConn1
  RR/RConn1 -- Subsystem3/RConn1

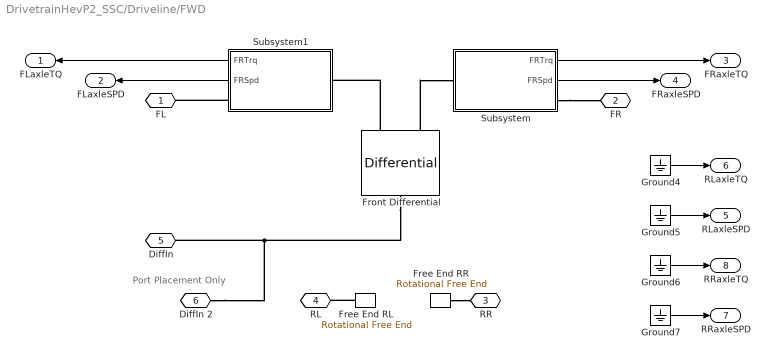
== system DrivetrainHevP2_SSC/Driveline/FWD ==
  note: Port Placement
      | Only
  Free End RL : fl_lib/Mechanical/Rotational Elements/Rotational Free End  w_specify=off  w_priority=None  w=0 rad/s  w_nominal_specify=off  w_nominal_unit=rad/s  w_nominal_value=1
      settings: SourceProductBaseCode=PW,SS,VE
  Free End RR : fl_lib/Mechanical/Rotational Elements/Rotational Free End  w_specify=off  w_priority=None  w=0 rad/s  w_nominal_specify=off  w_nominal_unit=rad/s  w_nominal_value=1
      settings: SourceProductBaseCode=PW,SS,VE
  Front Differential : sdl_lib/Gears/Differential  driveshaft_location=sdl.enum.differential_orientation.right  cd_ratio=FDrive  friction_model=sdl.enum.gear_friction.constant  efficiency=Eff_Diff  temperature_TLU=[ 280 300 320 ] K  efficiency_ss_TLU=[ 0.95 0.9 0.85 ]  efficiency_cd_TLU=[ 0.95 0.9 0.85 ]  pwr_thr=PwrThr_Diff W  mu_visc=VisFr_Diff N*m/(rad/s)  model_inertia=simscape.enum.onoff.on  carrier_inertia=JCa_Diff kg*m^2  planet_inertia=JPl_Diff kg*m^2  thermal_mass=50 J/K  T_init=300 K
      settings: SourceProductBaseCode=LD
  Ground{4..7} (4 alike) : Ground
  Subsystem : Subsystem
  Subsystem1 : Subsystem
  FL : PMIOPort  Side=Left
  FR : PMIOPort  Port=2  Side=Right
  RR : PMIOPort  Port=3  Side=Right
  RL : PMIOPort  Port=4  Side=Left
  DiffIn : PMIOPort  Port=5  Side=Left
  DiffIn 2 : PMIOPort  Port=6  Side=Right
  FLaxleTQ : Outport
  FLaxleSPD : Outport  Port=2
  FRaxleTQ : Outport  Port=3
  FRaxleSPD : Outport  Port=4
  RLaxleSPD : Outport  Port=5
  RLaxleTQ : Outport  Port=6
  RRaxleSPD : Outport  Port=7
  RRaxleTQ : Outport  Port=8
  wires:
  Subsystem1/1(FRTrq) -> FLaxleTQ/1
  Subsystem1/2(FRSpd) -> FLaxleSPD/1
  Subsystem/1(FRTrq) -> FRaxleTQ/1
  Subsystem/2(FRSpd) -> FRaxleSPD/1
  Ground5/1 -> RLaxleSPD/1
  Ground6/1 -> RRaxleTQ/1
  Ground7/1 -> RRaxleSPD/1
  Ground4/1 -> RLaxleTQ/1
  connections:
  Front Differential/LConn1 -- DiffIn 2/RConn1 -- DiffIn/RConn1
  Free End RR/LConn1 -- RR/RConn1
  Free End RL/LConn1 -- RL/RConn1
  Front Differential/RConn1 -- Subsystem1/LConn1
  Subsystem1/RConn1 -- FL/RConn1
  Front Differential/RConn2 -- Subsystem/LConn1
  Subsystem/RConn1 -- FR/RConn1

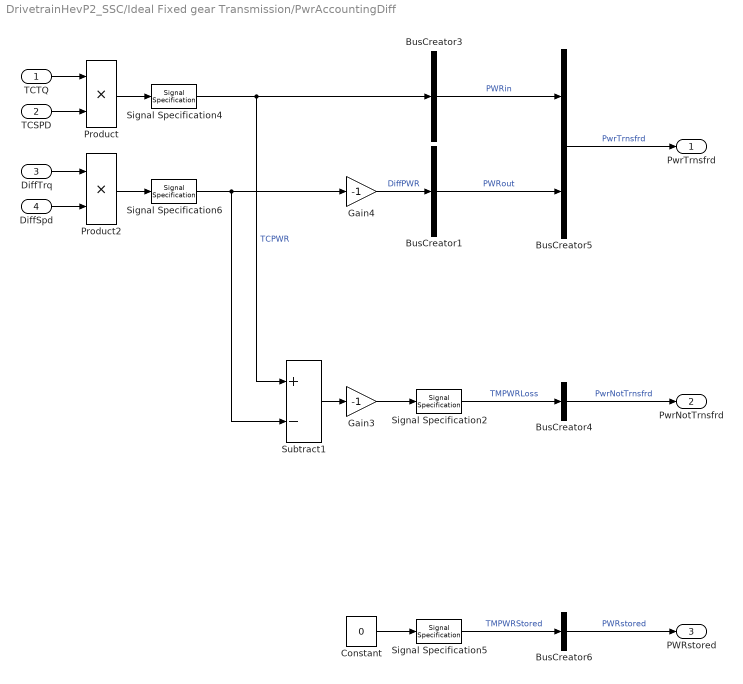
== system DrivetrainHevP2_SSC/Ideal Fixed gear Transmission/PwrAccountingDiff ==
  TCTQ : Inport
  TCSPD : Inport  Port=2
  DiffTrq : Inport  Port=3
  DiffSpd : Inport  Port=4
  BusCreator{1,3..4,6} (4 alike) : BusCreator  Inputs=1
  BusCreator5 : BusCreator  Inputs=2
  Constant : Constant  Value=0
  Gain3 : Gain  Gain=-1
  Gain4 : Gain  Gain=-1
  Product : Product
  Product2 : Product
  Signal Specification{2,4..6} (4 alike) : SignalSpecification  Unit=W
  Subtract1 : Sum  Inputs=+-
  PwrTrnsfrd : Outport
  PwrNotTrnsfrd : Outport  Port=2
  PWRstored : Outport  Port=3
  wires:
  Constant/1 -> Signal Specification5/1
  Product/1 -> Signal Specification4/1
  TCTQ/1 -> Product/1
  Product2/1 -> Signal Specification6/1
  Signal Specification2/1 -> BusCreator4/1  "TMPWRLoss"
  DiffSpd/1 -> Product2/2
  Gain3/1 -> Signal Specification2/1
  BusCreator3/1 -> BusCreator5/1  "PWRin"
  Signal Specification4/1 -> Subtract1/1, BusCreator3/1  "TCPWR"
  BusCreator1/1 -> BusCreator5/2  "PWRout"
  Signal Specification5/1 -> BusCreator6/1  "TMPWRStored"
  Signal Specification6/1 -> Subtract1/2, Gain4/1
  Subtract1/1 -> Gain3/1
  Gain4/1 -> BusCreator1/1  "DiffPWR"
  BusCreator4/1 -> PwrNotTrnsfrd/1  "PwrNotTrnsfrd"
  TCSPD/1 -> Product/2
  DiffTrq/1 -> Product2/1
  BusCreator6/1 -> PWRstored/1  "PWRstored"
  BusCreator5/1 -> PwrTrnsfrd/1  "PwrTrnsfrd"

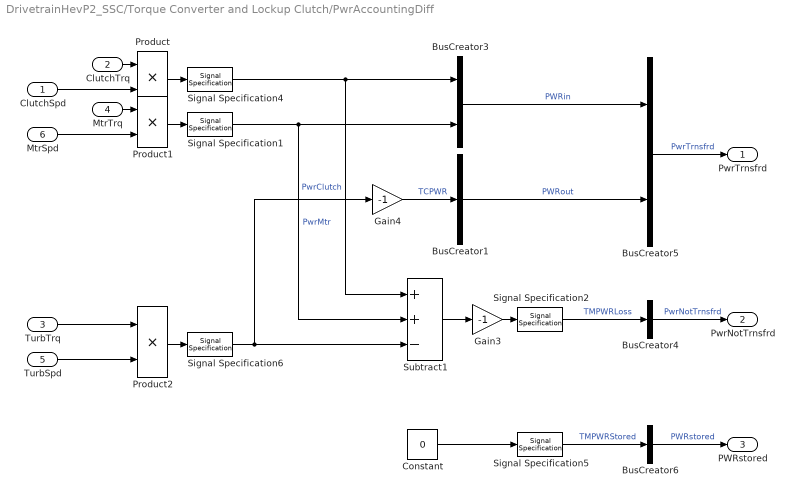
== system DrivetrainHevP2_SSC/Torque Converter and Lockup Clutch/PwrAccountingDiff ==
  ClutchSpd : Inport
  ClutchTrq : Inport  Port=2
  TurbTrq : Inport  Port=3
  MtrTrq : Inport  Port=4
  TurbSpd : Inport  Port=5
  MtrSpd : Inport  Port=6
  BusCreator1 : BusCreator  Inputs=1
  BusCreator3 : BusCreator  Inputs=2
  BusCreator4 : BusCreator  Inputs=1
  BusCreator5 : BusCreator  Inputs=2
  BusCreator6 : BusCreator  Inputs=1
  Constant : Constant  Value=0
  Gain3 : Gain  Gain=-1
  Gain4 : Gain  Gain=-1
  Product : Product
  Product1 : Product
  Product2 : Product
  Signal Specification{1..2,4..6} (5 alike) : SignalSpecification  Unit=W
  Subtract1 : Sum  Inputs=++-
  PwrTrnsfrd : Outport
  PwrNotTrnsfrd : Outport  Port=2
  PWRstored : Outport  Port=3
  wires:
  Constant/1 -> Signal Specification5/1
  Product/1 -> Signal Specification4/1
  TurbTrq/1 -> Product2/1
  Product2/1 -> Signal Specification6/1
  Signal Specification2/1 -> BusCreator4/1  "TMPWRLoss"
  Gain3/1 -> Signal Specification2/1
  BusCreator3/1 -> BusCreator5/1  "PWRin"
  Signal Specification4/1 -> Subtract1/1, BusCreator3/1  "PwrClutch"
  BusCreator1/1 -> BusCreator5/2  "PWRout"
  Signal Specification5/1 -> BusCreator6/1  "TMPWRStored"
  Signal Specification6/1 -> Gain4/1, Subtract1/3
  Subtract1/1 -> Gain3/1
  Gain4/1 -> BusCreator1/1  "TCPWR"
  BusCreator4/1 -> PwrNotTrnsfrd/1  "PwrNotTrnsfrd"
  TurbSpd/1 -> Product2/2
  BusCreator6/1 -> PWRstored/1  "PWRstored"
  BusCreator5/1 -> PwrTrnsfrd/1  "PwrTrnsfrd"
  ClutchTrq/1 -> Product/1
  MtrTrq/1 -> Product1/1
  ClutchSpd/1 -> Product/2
  MtrSpd/1 -> Product1/2
  Product1/1 -> Signal Specification1/1
  Signal Specification1/1 -> Subtract1/2, BusCreator3/2  "PwrMtr"

== system DrivetrainHevP2_SSC/Transmission/Actuator ==
  State : Inport
  Actuator dynamics : Subsystem  mask(First-order lag supporting vector signals){b=[1 1 1 1 1]*0.05, x_initial=1}
      mask prompts: b "Filter time constant"; x_initial "Initial output"
      mask help: Models a lag of the form 1/(b*s+1) where s is the Laplace operator.
  Demux : Demux  Outputs=5
  Simulink-PS Converter{,1..4} (5 alike) : nesl_utility/Simulink-PS Converter  PhysicalDomain=network_engine_domain  SubClassName=ps_input  LeftPortType=input  RightPortType=output  PseudoPeriodic=off  Frequencies=[]  NoiseDistribution=none  NoiseParameters=[]  Unit=1  AffineConversion=off  FilteringAndDerivatives=zero  SimscapeFilterOrder=1  InputFilterTimeConstant=0.001  UdotUserProvided=1
      settings: SourceProductBaseCode=SS,PW,VE
  State to pressure : Gain  Gain=[1e7, 1e7, 1e7, 1e7,1e7]
  Cl E : PMIOPort  Side=Right
  Cl A : PMIOPort  Port=2  Side=Right
  Cl D : PMIOPort  Port=3  Side=Right
  Cl B : PMIOPort  Port=4  Side=Right
  Cl C : PMIOPort  Port=5  Side=Right
  wires:
  Demux/3 -> Simulink-PS Converter2/1
  Demux/5 -> Simulink-PS Converter4/1
  State to pressure/1 -> Demux/1
  Demux/4 -> Simulink-PS Converter3/1
  Demux/2 -> Simulink-PS Converter1/1
  Demux/1 -> Simulink-PS Converter/1
  Actuator dynamics/1(Out) -> State to pressure/1
  State/1 -> Actuator dynamics/1(In)
  connections:
  Simulink-PS Converter4/RConn1 -- Cl E/RConn1
  Simulink-PS Converter3/RConn1 -- Cl D/RConn1
  Simulink-PS Converter2/RConn1 -- Cl C/RConn1
  Simulink-PS Converter/RConn1 -- Cl A/RConn1
  Simulink-PS Converter1/RConn1 -- Cl B/RConn1

== system DrivetrainHevP2_SSC/Transmission/Clutch Schedule ==
  note: Gear
      | A
      | B
      | C
      | D
      | E
      | Ratio
      |
      | 6
      | 0
      | 1
      | 0
      | 0
      | 1
      | g2/(1+g2)
      |
      | 5
      | 1
      | 1
      | 0
      | 0
      | 0
      | g2/(g2+1/(1+g1))
      |
      | 4
      | 0
      | 1
      | 1
      | 0
      | 0
      | g3(1+g1)/(g3(1+g1)-1)
      |
      | 3
      | 1
      | 0
      | 1
      | 0
      | 0
      | (1+g1)/g1
      |
      | 2
      | 0
      | 0
      | 1
      | 0
      | 1
      | (1+g1)(g3+g2)/(g1(1+g2))
      |
      | 1
      | 0
      | 0
      | 1
      | 1
      | 0
      | g3(1+g1)/g1
      |
      | R
      | 1
      | 0
      | 0
      | 1
      | 0
      | -g2(1+g1)/g1
  note: g1: Planetary ring/sun gear ratio
      | g2: Ravigneaux ring/large sun gear ratio
      | g3: Ravigneaux ring/small sun gear ratio
  note: 0 - Disengaged, 1 - Engaged
  note: Clutch Schedule
  Gear : Inport
  Constant : Constant  Value=[0 0 1 1 0]
  Constant1 : Constant  Value=[1 0 0 1 0]
  Constant2 : Constant  Value=[0 0 1 1 0]
  Constant3 : Constant  Value=[0 0 1 0 1]
  Constant4 : Constant  Value=[1 0 1 0 0]
  Constant5 : Constant  Value=[0 1 1 0 0]
  Constant6 : Constant  Value=[1 1 0 0 0]
  Constant7 : Constant  Value=[0 1 0 0 1]  VectorParams1D=off
  Rounding Function : Rounding
  Saturation : Saturate  UpperLimit=6  LowerLimit=-1  ZeroCross=off
  Select Clutch States : MultiPortSwitch  DataPortOrder=Specify indices  DataPortIndices={6,5,4,3,2,1,-1,0}  DiagnosticForDefault=None  SaturateOnIntegerOverflow=off  InputSameDT=off
  St : Outport  VectorParamsAs1DForOutWhenUnconnected=off
  wires:
  Select Clutch States/1 -> St/1
  Gear/1 -> Saturation/1
  Constant/1 -> Select Clutch States/9
  Saturation/1 -> Rounding Function/1
  Rounding Function/1 -> Select Clutch States/1
  Constant1/1 -> Select Clutch States/8
  Constant2/1 -> Select Clutch States/7
  Constant3/1 -> Select Clutch States/6
  Constant4/1 -> Select Clutch States/5
  Constant5/1 -> Select Clutch States/4
  Constant6/1 -> Select Clutch States/3
  Constant7/1 -> Select Clutch States/2

== system DrivetrainHevP2_SSC/Transmission/Efficiency ==
  Pout : Inport
  PIn : Inport  Port=2
  Divide1 : Product  Inputs=*/
  Mux : Mux  Inputs=2
  Saturation : Saturate  UpperLimit=100  LowerLimit=0.1  ZeroCross=off
  Saturation1 : Saturate  UpperLimit=100  LowerLimit=-100  ZeroCross=off
  Terminator : Terminator
  Terminator1 : Terminator
  wires:
  Saturation/1 -> Mux/2, Divide1/2  "power_in"
  Saturation1/1 -> Mux/1, Divide1/1  "power_out"
  Divide1/1 -> Terminator1/1  "efficiency"
  Mux/1 -> Terminator/1
  PIn/1 -> Saturation/1
  Pout/1 -> Saturation1/1

== system DrivetrainHevP2_SSC/Transmission/R ==
  Ideal Rotational Motion Sensor : fl_lib/Mechanical/Mechanical Sensors/Ideal Rotational Motion Sensor  wrap_angle=simscape.enum.onoff.off  offset=0 rad
      settings: SourceProductBaseCode=PW,SS,VE
  MRRef Brake C4 : fl_lib/Mechanical/Rotational Elements/Mechanical Rotational Reference
      settings: SourceProductBaseCode=PW,SS,VE
  PS-Simulink Converter : nesl_utility/PS-Simulink Converter  PhysicalDomain=network_engine_domain  SubClassName=ps_output  LeftPortType=input  RightPortType=output  PseudoPeriodic=off  Frequencies=[]  VectorFormat=1-D array  Unit=1  AffineConversion=off
      settings: SourceProductBaseCode=SS,PW,VE
  Terminator : Terminator
  B : PMIOPort  Side=Left
  tag scope: w_in=global
  wires:
  PS-Simulink Converter/1 -> [w_in], Terminator/1  "win_ssc"
  connections:
  PS-Simulink Converter/LConn1 -- Ideal Rotational Motion Sensor/RConn2
  MRRef Brake C4/LConn1 -- Ideal Rotational Motion Sensor/RConn1
  Ideal Rotational Motion Sensor/LConn1 -- B/RConn1

== system DrivetrainHevP2_SSC/Transmission/R2 ==
  Ideal Rotational Motion Sensor : fl_lib/Mechanical/Mechanical Sensors/Ideal Rotational Motion Sensor  wrap_angle=simscape.enum.onoff.off  offset=0 rad
      settings: SourceProductBaseCode=PW,SS,VE
  MRRef Brake C4 : fl_lib/Mechanical/Rotational Elements/Mechanical Rotational Reference
      settings: SourceProductBaseCode=PW,SS,VE
  PS-Simulink Converter : nesl_utility/PS-Simulink Converter  PhysicalDomain=network_engine_domain  SubClassName=ps_output  LeftPortType=input  RightPortType=output  PseudoPeriodic=off  Frequencies=[]  VectorFormat=1-D array  Unit=1  AffineConversion=off
      settings: SourceProductBaseCode=SS,PW,VE
  Terminator : Terminator
  B : PMIOPort  Side=Left
  tag scope: w_out=global
  wires:
  PS-Simulink Converter/1 -> [w_out], Terminator/1  "wout_ssc"
  connections:
  Ideal Rotational Motion Sensor/LConn1 -- B/RConn1
  MRRef Brake C4/LConn1 -- Ideal Rotational Motion Sensor/RConn1
  PS-Simulink Converter/LConn1 -- Ideal Rotational Motion Sensor/RConn2
